simulink model "Major_project"  (Simulink 7.3)
settings: Solver=ode45  StartTime=0.0  StopTime=10  RelTol=1e-3
libraries: powerlib x13, powerlib_extras x2, spsUniversalBridgeModel x1
settings Model: Creator=win7  LastModifiedBy=win7

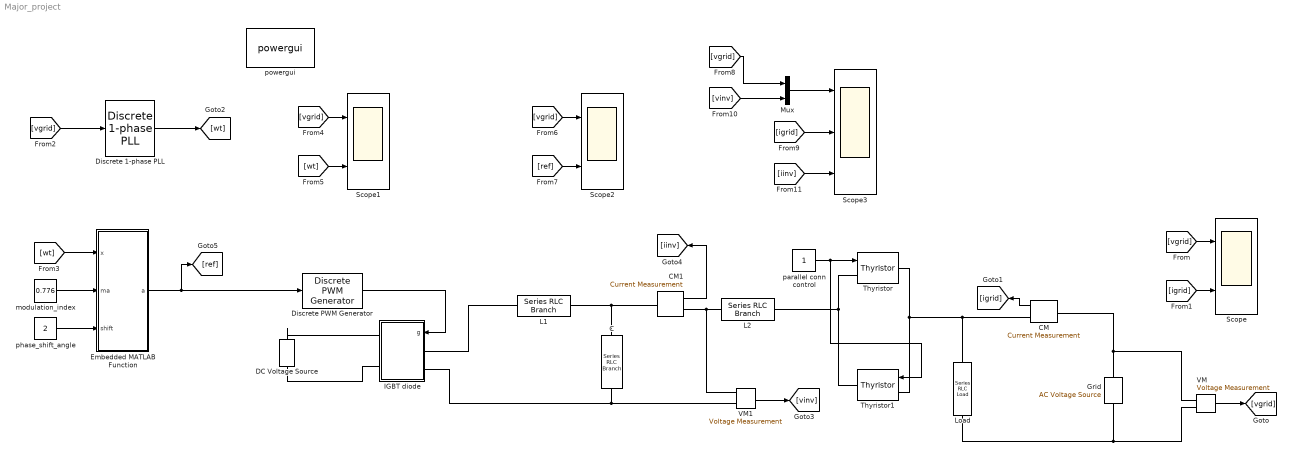
== system Major_project ==
  C : powerlib/Elements/Series RLC Branch  DialogController=POWERSYS.PowerSysDialog  PhysicalDomain=powersysdomain  SubClassName=unknown  LeftPortType=p1  RightPortType=p1  LConnTagsString=__new0  RConnTagsString=__new0  BranchType=RC  Resistance=0.1  Inductance=1e-3  SetiL0=off  InitialCurrent=0  Capacitance=10e-6  Setx0=off  InitialVoltage=0  Measurements=None
  CM : powerlib/Measurements/Current Measurement  DialogController=POWERSYS.PowerSysDialog  SystemSampleTime=-1  PhasorSimulation=off  OutputType=Complex  PSBequivalent=0
  CM1 : powerlib/Measurements/Current Measurement  DialogController=POWERSYS.PowerSysDialog  SystemSampleTime=-1  PhasorSimulation=off  OutputType=Complex  PSBequivalent=0
  DC Voltage Source : powerlib/Electrical Sources/DC Voltage Source  DialogController=POWERSYS.PowerSysDialog  SystemSampleTime=-1  Amplitude=400  Measurements=None
  Discrete 1-phase PLL : powerlib_extras/Discrete  Control Blocks/Discrete 1-phase PLL  SystemSampleTime=-1  Fmin=45  Par_Init=[0 50]  ParK=[ 180 3200 1]  Ts=1e-4  AGC=off
  Discrete PWM Generator : powerlib_extras/Discrete  Control Blocks/Discrete PWM Generator  DialogController=POWERSYS.PowerSysDialog  SystemSampleTime=-1  GeneratorMode="2-arm  bridge (4 pulses)"  Fc=3000  Ts=5e-6  Internal=off  mIndex=0.4  Freq=60  Phase=1
  Embedded MATLAB Function : Stateflow chart
  Grid : powerlib/Electrical Sources/AC Voltage Source  DialogController=POWERSYS.PowerSysDialog  SystemSampleTime=-1  Amplitude=220*sqrt(2)  Phase=0  Frequency=50  SampleTime=1e-5  Measurements=None
  IGBT diode : Subsystem  AncestorBlock=powerlib/Power Electronics/Universal Bridge  DialogController=POWERSYS.PowerSysDialog  mask(Universal Bridge){Arms=2, SnubberResistance=1e5, SnubberCapacitance=inf, Device=IGBT / Diodes, Ron=1e-3, Lon=0, ForwardVoltages=[  0  0  ], ForwardVoltage=0, GTOparameters=[ 10e-6 , 20e-6 ], IGBTparameters=[ 1e-6 , 2e-6 ], Measurements=None, Measurements_2=None, converterType=Rectifier}
      mask prompts: Arms "Number of bridge arms:"; SnubberResistance "Snubber resistance Rs (Ohms)"; SnubberCapacitance "Snubber capacitance Cs (F)"; Device "Power Electronic device"; Ron "Ron (Ohms)"; Lon "Lon (H)"; ForwardVoltages "Forward voltages  [ Device Vf(V) , Diode Vfd(V)]"; ForwardVoltage "Forward voltage Vf (V)"; GTOparameters "[  Tf (s) , Tt (s)  ]"; IGBTparameters "[  Tf (s) , Tt (s)  ]"; Measurements_2 "Measurements"; converterType "Converter type:"
      mask help: This block implement a bridge of selected power electronics devices. Series RC snubber circuits are connected in parallel with each switch device. Press Help for suggested snubber values when the model is discretized. For most applications the internal inductance Lon of diodes and thyristors should be set to zero
      mask init:
      | block = gcb;
      | [WantBlockChoice,Ts,Switches,Tf_sps,Tt_sps,Vf,Vf_SwitchOn,Vf_DiodeOn,IC,SignalLength,ReorderGatesDelays,X,Y,Ron] = powericon('UniversalBridgeInit',block,Device,Arms,ForwardVoltage,ForwardVoltages,GTOparameters,IGBTparameters,Ron);
      | powericon('SetInternalModels','set',block,WantBlockChoice);
      settings: CopyFcn=powericon('SwitchesCopyFcn','Universal Bridge',gcb)
      mask Help: web(psbhelp);
      mask StyleString: popup(1|2|3),edit,edit,popup(Diodes|Thyristors|GTO / Diodes|MOSFET / Diodes|IGBT / Diodes|Ideal Switches|Switching-function based VSC|Average-model based VSC),edit,edit,edit,edit,edit,edit,popup(None|Device voltages|Device currents|UAB UBC UCA UDC voltages|All voltages and currents),popup(None|Voltages|Currents|Voltages and Currents),popup(Rectifier|Inverter)
      mask CallbackString: powericon('UniversalBridgeCback',gcb);|||powericon('UniversalBridgeCback',gcb);|||||||||
      mask Display: plot(0,0,100,100,X.p1,Y.p1,X.p2,Y.p2,X.p3,Y.p3,X.p4,Y.p4,X.p5,Y.p5,X.p6,Y.p6,X.p7,Y.p7);
  L1 : powerlib/Elements/Series RLC Branch  DialogController=POWERSYS.PowerSysDialog  PhysicalDomain=powersysdomain  SubClassName=unknown  LeftPortType=p1  RightPortType=p1  LConnTagsString=__new0  RConnTagsString=__new0  BranchType=L  Resistance=1  Inductance=17.7e-4  SetiL0=off  InitialCurrent=0  Capacitance=1e-6  Setx0=off  InitialVoltage=0  Measurements=None
  L2 : powerlib/Elements/Series RLC Branch  DialogController=POWERSYS.PowerSysDialog  PhysicalDomain=powersysdomain  SubClassName=unknown  LeftPortType=p1  RightPortType=p1  LConnTagsString=__new0  RConnTagsString=__new0  BranchType=L  Resistance=1  Inductance=5.7e-4  SetiL0=off  InitialCurrent=0  Capacitance=1e-6  Setx0=off  InitialVoltage=0  Measurements=None
  Load : powerlib/Elements/Series RLC Load  DialogController=POWERSYS.PowerSysDialog  PhysicalDomain=powersysdomain  SubClassName=unknown  LeftPortType=p1  RightPortType=p1  LConnTagsString=a  RConnTagsString=__new0  NominalVoltage=220  NominalFrequency=50  ActivePower=220*10/sqrt(2)  InductivePower=220*1/sqrt(2)  CapacitivePower=0  Setx0=off  InitialVoltage=0  SetiL0=off  InitialCurrent=0  Measurements=None
  Mux : Mux  Inputs=2
  Scope : Scope  NumInputPorts=2
      settings: TickLabels=on  TimeRange=0.09  YMin=-350~-11  YMax=350~11
  Scope1 : Scope  NumInputPorts=2
      settings: TickLabels=on  TimeRange=0.09  YMin=-350~0  YMax=350~6.5
  Scope2 : Scope  NumInputPorts=2
      settings: TickLabels=on  TimeRange=0.09  YMin=-350~-0.8  YMax=350~0.8  SaveName=ScopeData2
  Scope3 : Scope  NumInputPorts=3
      settings: TickLabels=on  TimeRange=0.1  YMin=-350~-12.5~-8e-016  YMax=350~12.5~8e-016  SaveName=ScopeData3
  Thyristor : powerlib/Power Electronics/Thyristor  DialogController=POWERSYS.PowerSysDialog  SystemSampleTime=-1  Ron=0.001  Lon=0  Vf=0.8  IC=0  Rs=500  Cs=250e-9  Measurements=off
  Thyristor1 : powerlib/Power Electronics/Thyristor  DialogController=POWERSYS.PowerSysDialog  SystemSampleTime=-1  Ron=0.001  Lon=0  Vf=0.8  IC=0  Rs=500  Cs=250e-9  Measurements=off
  VM : powerlib/Measurements/Voltage Measurement  DialogController=POWERSYS.PowerSysDialog  SystemSampleTime=-1  PhasorSimulation=off  OutputType=Complex  PSBequivalent=0
  VM1 : powerlib/Measurements/Voltage Measurement  DialogController=POWERSYS.PowerSysDialog  SystemSampleTime=-1  PhasorSimulation=off  OutputType=Complex  PSBequivalent=0
  modulation_index : Constant  Value=0.776  OutDataType=fixdt(1, 16)  OutScaling=2^0
  parallel conn control : Constant  OutDataType=fixdt(1, 16)  OutScaling=2^0
  phase_shift_angle : Constant  Value=2  OutDataType=fixdt(1, 16)  OutScaling=2^0
  powergui : powerlib/powergui  Priority=1  SystemSampleTime=-1  SimulationMode=Discrete  SampleTime=1e-06  frequency=60  SPID=off  DisableSnubberDevices=off  DisableRonSwitches=off  DisableVfSwitches=off  SwTol=0  Interpol=off  frequencyindice=50  echomessages=off  HookPort=off  DisplayEquations=off  FunctionMessages=off  EnableUseOfTLC=off  x0status=blocks  RestoreLinks=warning  Frange=[0:2:500]  Ylog=off  Xlog=on  ShowGrid=off  save=off  variable=ZData  ZoomFFT=on  StartTime=0.0  cycles=1  DisplayStyle=1  fundamental=60  FreqAxis=off  MaxFrequency=1000  frequencyindicesteady=1  RmsSteady=1  display=off  Ts=0  methode=off
  wires:
  VM/1 -> [vgrid]
  [vgrid] -> Scope/1
  CM/1 -> [igrid]
  [igrid] -> Scope/2
  [vgrid] -> Discrete 1-phase PLL/1
  Discrete 1-phase PLL/2 -> [wt]
  Discrete PWM Generator/1 -> IGBT diode/1(g)
  Embedded MATLAB Function/1(a) -> Discrete PWM Generator/1, [ref]
  modulation_index/1 -> Embedded MATLAB Function/2(ma)
  phase_shift_angle/1 -> Embedded MATLAB Function/3(shift)
  [wt] -> Embedded MATLAB Function/1(x)
  [vgrid] -> Scope1/1
  [wt] -> Scope1/2
  VM1/1 -> [vinv]
  CM1/1 -> [iinv]
  [vgrid] -> Scope2/1
  [ref] -> Scope2/2
  [igrid] -> Scope3/2
  Mux/1 -> Scope3/1
  [vgrid] -> Mux/1
  [vinv] -> Mux/2
  [iinv] -> Scope3/3
  parallel conn control/1 -> Thyristor/1, Thyristor1/1
  connections:
  Grid/RConn1 -- VM/LConn1 -- CM/LConn1
  Load/RConn1 -- VM/LConn2 -- Grid/LConn1
  CM/RConn1 -- Load/LConn1 -- Thyristor/RConn1 -- Thyristor1/LConn1
  DC Voltage Source/LConn1 -- IGBT diode/RConn2
  DC Voltage Source/RConn1 -- IGBT diode/RConn1
  IGBT diode/LConn1 -- L1/LConn1
  C/LConn1 -- L1/RConn1 -- CM1/LConn1
  C/RConn1 -- IGBT diode/LConn2 -- VM1/LConn2
  CM1/RConn1 -- L2/LConn1 -- VM1/LConn1
  Thyristor1/RConn1 -- L2/RConn1 -- Thyristor/LConn1

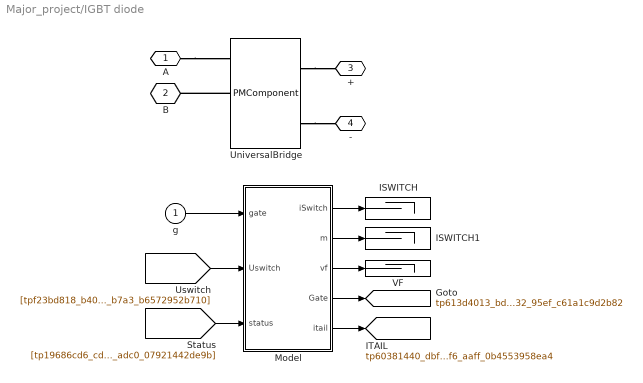
== system Major_project/IGBT diode ==
  g : Inport
  ISWITCH : Terminator
  ISWITCH1 : Terminator
  Model : Subsystem  BlockChoice=discrete IGBT
      settings: AttributesFormatString=%<BlockChoice>  TemplateBlock=spsUniversalBridgeModel/model  MemberBlocks=SPID,continuous Average model 1,continuous Average model 2,continuous Average model 3,continuous Diode-Logic,continuous Diode-RL,continuous GTO,continuous IGBT,continuous Ideal Switch,continuous MOSFET,continuous Switching function 1,continuous Switching function 2,continuous Switching function 3,continuous Thyristor-Logic,continuous Thyristor-RL,discrete Average model 1,discrete Average model 2,discrete Average model 3,discrete Diode-Logic,discrete GTO,discrete IGBT,discrete Ideal Switch,discrete MOSFET,discrete Switching function 1,discrete Switching function 2,discrete Switching function 3,discrete Thyristor-Logic
      mask Display: disp('Template')
  UniversalBridge : PMComponent  PhysicalDomain=powersysdomain  LeftPortType=p1  RightPortType=p1  LConnTagsString=A|B|C  RConnTagsString=+|-
      mask Type: InnerPowersysBlock
  VF : Terminator
  A : PMIOPort  Port=1  Side=Left
  B : PMIOPort  Port=2  Side=Left
  + : PMIOPort  Port=3  Side=Right
  - : PMIOPort  Port=4  Side=Right
  tag scope: tp60381440_dbfd_47f6_aaff_0b4553958ea4=global, tp613d4013_bd6b_4432_95ef_c61a1c9d2b82=global
  wires:
  g/1 -> Model/1(gate)
  [tpf23bd818_b406_453e_b7a3_b6572952b710] -> Model/2(Uswitch)
  [tp19686cd6_cd07_4bd5_adc0_07921442de9b] -> Model/3(status)
  Model/4(Gate) -> [tp613d4013_bd6b_4432_95ef_c61a1c9d2b82]
  Model/3(vf) -> VF/1
  Model/5(itail) -> [tp60381440_dbfd_47f6_aaff_0b4553958ea4]
  Model/1(iSwitch) -> ISWITCH/1
  Model/2(m) -> ISWITCH1/1
  connections:
  UniversalBridge/LConn2 -- B/RConn1
  UniversalBridge/RConn2 -- -/RConn1
  UniversalBridge/RConn1 -- +/RConn1
  A/RConn1 -- UniversalBridge/LConn1

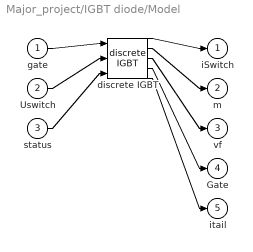
== system Major_project/IGBT diode/Model ==
  gate : Inport  OutDataType=sfix(16)  OutScaling=2^0
  Uswitch : Inport  Port=2  OutDataType=sfix(16)  OutScaling=2^0
  status : Inport  Port=3  OutDataType=sfix(16)  OutScaling=2^0
  discrete IGBT : spsUniversalBridgeModel/discrete IGBT  SystemSampleTime=-1
  iSwitch : Outport  OutDataType=sfix(16)  OutScaling=2^0
  m : Outport  Port=2  OutDataType=sfix(16)  OutScaling=2^0
  vf : Outport  Port=3  OutDataType=sfix(16)  OutScaling=2^0
  Gate : Outport  Port=4  OutDataType=sfix(16)  OutScaling=2^0
  itail : Outport  Port=5  OutDataType=sfix(16)  OutScaling=2^0
  wires:
  gate/1 -> discrete IGBT/1
  Uswitch/1 -> discrete IGBT/2
  status/1 -> discrete IGBT/3
  discrete IGBT/1 -> iSwitch/1
  discrete IGBT/2 -> m/1
  discrete IGBT/3 -> vf/1
  discrete IGBT/4 -> Gate/1
  discrete IGBT/5 -> itail/1

== matlab function Embedded MATLAB Function ==
  data: x input double; a output double; ma input double; shift input double
function a = fcn(x,ma,shift)
shift_k=shift*pi/180;
a = (ma*(sin((x)+shift_k)));
